simulink model "VIM_simu"  (R2022b)
settings: Solver=VariableStepAuto  StartTime=0.0  StopTime=0.7  MaxStep=1e-4  RelTol=1e-3
undefined symbols (not defined in the file or in its folder): motorParams, params_struct_torque
libraries: slpidlib x6, spsabctodq0Lib x6, spsdq0toabcLib x2, spsThreePhaseSeriesRLCBranchLib x2, spsThreePhaseSeriesRLCLoadLib x2, spsThreePhaseVIMeasurementLib x2, spsDCVoltageSourceLib x1, spsGroundLib x1, spsPower3phInstantaneousLib x1, spsPWMGenerator2LevelLib x1, spsThreePhaseBreakerLib x1, spsThreePhaseSourceLib x1
settings Model: Creator=Dong  LastModifiedBy=Dong
settings DebuggingCC: MaskedZcDiagnostic=none  IgnoredZcDiagnostic=none

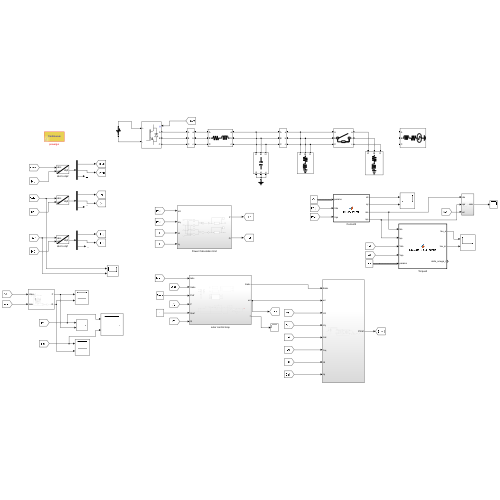
[thumbnail: Simulink's stored preview of the top-level diagram]
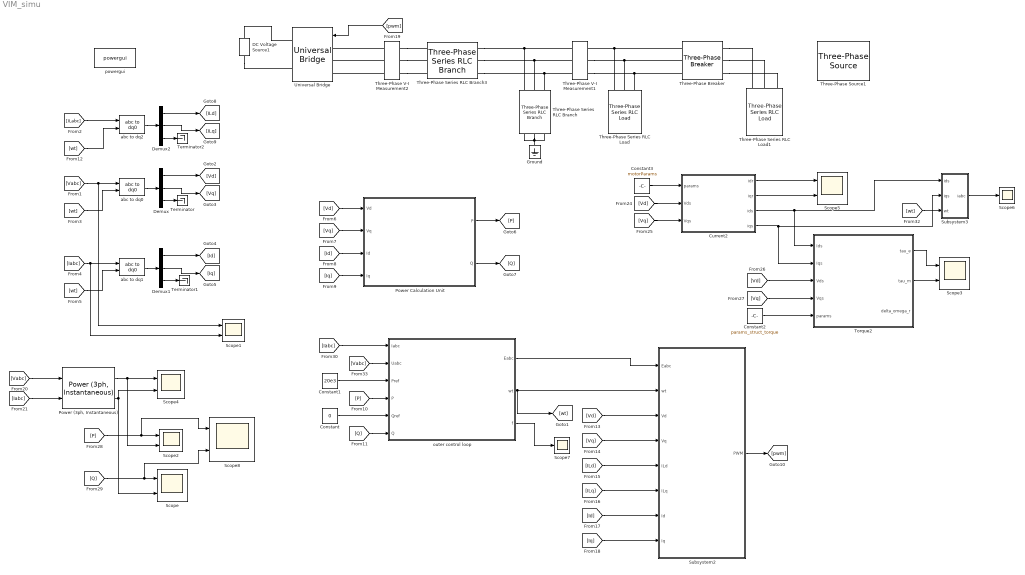
== system VIM_simu ==
  Constant : Constant  Value=0
  Constant1 : Constant  Value=20e3
  Constant2 : Constant  Value=params_struct_torque  OutDataTypeStr=Bus: paramsBusTorque
  Constant3 : Constant  Value=motorParams  OutDataTypeStr=Bus: motorParamsBus
  Current2 : MATLAB Function  TreatAsAtomicUnit=on
  DC Voltage Source1 : spsDCVoltageSourceLib/DC Voltage Source  Amplitude=800  Measurements=None
  Demux : Demux  Outputs=3
  Demux1 : Demux  Outputs=3
  Demux2 : Demux  Outputs=3
  Ground : spsGroundLib/Ground  LConnTagsString=a
  "Power (3ph, Instantaneous)" : spsPower3phInstantaneousLib/Power (3ph, Instantaneous)
  Power Calculation Unit : Subsystem
  Scope{,1..5,8} (7 alike) : Scope  NumInputPorts=2
  Scope6 : Scope
  Scope7 : Scope
  Subsystem2 : Subsystem
  Subsystem3 : Subsystem
  Terminator : Terminator
  Terminator1 : Terminator
  Terminator2 : Terminator
  Three-Phase Series RLC Branch : spsThreePhaseSeriesRLCBranchLib/Three-Phase Series RLC Branch  LConnTagsString=A|B|C  RConnTagsString=A|B|C  BranchType=C  Resistance=1e-5  Inductance=3e-3  Capacitance=40e-6  Measurements=None
  Three-Phase Series RLC Branch3 : spsThreePhaseSeriesRLCBranchLib/Three-Phase Series RLC Branch  LConnTagsString=A|B|C  RConnTagsString=A|B|C  BranchType=RL  Resistance=1e-5  Inductance=3e-3  Capacitance=1e-6  Measurements=None
  Three-Phase Series RLC Load : spsThreePhaseSeriesRLCLoadLib/Three-Phase Series RLC Load  LConnTagsString=A|B|C  Configuration=Y (grounded)  NominalVoltage=380  Vabc=[1e3 1e3 1e3]  Vabcp=[1e3 1e3 1e3]  NominalFrequency=50  UnbalancedPower=off  ActivePower=5e3  InductivePower=200  CapacitivePower=0  Pabc=[10e3 9e3 11e3]  QLabc=[100 90 110]  QCabc=[100 90 110]  Pabcp=[10e3 9e3 11e3]  QLabcp=[100 90 110]  QCabcp=[100 90 110]  Measurements=None  LoadType=constant Z
  Three-Phase Series RLC Load1 : spsThreePhaseSeriesRLCLoadLib/Three-Phase Series RLC Load  LConnTagsString=A|B|C  Configuration=Y (grounded)  NominalVoltage=380  Vabc=[1e3 1e3 1e3]  Vabcp=[1e3 1e3 1e3]  NominalFrequency=50  UnbalancedPower=off  ActivePower=5e3  InductivePower=500  CapacitivePower=0  Pabc=[10e3 9e3 11e3]  QLabc=[100 90 110]  QCabc=[100 90 110]  Pabcp=[10e3 9e3 11e3]  QLabcp=[100 90 110]  QCabcp=[100 90 110]  Measurements=None  LoadType=constant Z
  Three-Phase V-I Measurement1 : spsThreePhaseVIMeasurementLib/Three-Phase V-I Measurement  VoltageMeasurement=phase-to-ground  SetLabelV=on  LabelV=Vabc  Vpu=off  VpuLL=off  CurrentMeasurement=yes  SetLabelI=on  LabelI=Iabc  Ipu=off  Pbase=100e6  Vbase=500e3  OutputType=Complex  PhasorSimulation=off  PSBequivalent=0
  Three-Phase V-I Measurement2 : spsThreePhaseVIMeasurementLib/Three-Phase V-I Measurement  VoltageMeasurement=no  SetLabelV=off  LabelV=Vabc  Vpu=off  VpuLL=off  CurrentMeasurement=yes  SetLabelI=on  LabelI=ILabc  Ipu=off  Pbase=100e6  Vbase=500e3  OutputType=Complex  PhasorSimulation=off  PSBequivalent=0
  Three-Phase Breaker : spsThreePhaseBreakerLib/Three-Phase Breaker  InitialState=open  SwitchA=on  SwitchB=on  SwitchC=on  SwitchTimes=[0.1 0.4]  External=off  BreakerResistance=0.01  SnubberResistance=1e6  SnubberCapacitance=inf  Measurements=None
  Three-Phase Source1 : spsThreePhaseSourceLib/Three-Phase Source  InternalConnection=Yg  VoltagePhases=off  Voltage=380  PhaseAngle=0  Voltage_phases=[25e3 25e3 25e3]/sqrt(3)  PhaseAngles_phases=[0 -120 +120]  Frequency=50  NonIdealSource=on  SpecifyImpedance=off  Resistance=1e-4  Inductance=1e-3  ShortCircuitLevel=100e6  BaseVoltage=25e3  XRratio=7  BusType=swing  Pref=10e3  Qref=0  Prefabc=[10e3, 10e3, 10e3]  Qrefabc=[0, 0, 0]  Qmin=-inf  Qmax=inf
  Torque2 : MATLAB Function  TreatAsAtomicUnit=on
  Universal Bridge : spsUniversalBridgeLib/Universal Bridge  Arms=3  SnubberResistance=1e5  SnubberCapacitance=inf  Device=IGBT / Diodes  Ron=1e-3  Lon=0  ForwardVoltages="[  0  0  ]"  ForwardVoltage=0  GTOparameters=[ 10e-6 , 20e-6 ]  IGBTparameters=[ 1e-6 , 2e-6 ]  Measurements=None  Measurements_2=None  converterType=Rectifier
  abc to dq0 : spsabctodq0Lib/abc to dq0  Alignment=90 degrees behind phase A axis
  abc to dq1 : spsabctodq0Lib/abc to dq0  Alignment=90 degrees behind phase A axis
  abc to dq2 : spsabctodq0Lib/abc to dq0  Alignment=90 degrees behind phase A axis
  outer control loop : Subsystem
  powergui : sps_lib/powergui  Priority=1  SimulationMode=Continuous  SampleTime=50e-6  frequency=60  Iterations=50  frequencyindice=0  Pbase=100e6  ErrMax=1e-4  UnitsV=kV  UnitsW=MW  buscounter=0  FunctionMessages=off  echomessages=off  EnableUseOfTLC=off  CurrentSourceSwitches=off  DisableSnubberDevices=off  DisableRonSwitches=off  DisableVfSwitches=off  DisplayEquations=off  AutomaticDiscreteSolvers=off  SolverType=Tustin/Backward Euler (TBE)  Interpol=off  ExternalGateDelay=off  methode=off  Ts=100  x0status=blocks  SPID=on  SwTol=0  HookPort=off  NonlinearTolerance=1e-4  nMaxIteration=100  ContinueOnMaxIteration=off  RestoreLinks=warning  ResistiveCurrentMeasurement=off  Frange=[0:2:500]  Ylog=off  Xlog=on  ShowGrid=off  save=off  variable=ZData  structure=0  ZoomFFT=off  StartTime=0.0  cycles=1  DisplayStyle=1  fundamental=60  FreqAxis=off  MaxFrequency=1000  frequencyindicesteady=1  RmsSteady=1  display=off
  wires:
  Constant/1 -> outer control loop/5(Qref)
  Constant1/1 -> outer control loop/3(Pref)
  [Vabc] -> abc to dq0/1, Scope1/1
  [wt] -> abc to dq0/2
  [wt] -> abc to dq1/2
  [Iabc] -> Scope1/2, abc to dq1/1
  abc to dq0/1 -> Demux/1
  abc to dq1/1 -> Demux1/1
  Demux1/3 -> Terminator1/1
  Demux/3 -> Terminator/1
  Demux/1 -> [Vd]
  Demux/2 -> [Vq]
  Demux1/2 -> [Iq]
  Demux1/1 -> [Id]
  [Vd] -> Power Calculation Unit/1(Vd)
  [Vq] -> Power Calculation Unit/2(Vq)
  [Id] -> Power Calculation Unit/3(Id)
  [Iq] -> Power Calculation Unit/4(Iq)
  Power Calculation Unit/1(P) -> [P]
  Power Calculation Unit/2(Q) -> [Q]
  [P] -> outer control loop/4(P)
  [Q] -> outer control loop/6(Q)
  Demux2/2 -> [ILq]
  Demux2/1 -> [ILd]
  Demux2/3 -> Terminator2/1
  abc to dq2/1 -> Demux2/1
  [wt] -> abc to dq2/2
  [ILabc] -> abc to dq2/1
  outer control loop/1(Eabc) -> Subsystem2/1(Eabc)
  [Vd] -> Subsystem2/3(Vd)
  [Vq] -> Subsystem2/4(Vq)
  [ILd] -> Subsystem2/5(ILd)
  [ILq] -> Subsystem2/6(ILq)
  [Iq] -> Subsystem2/8(Iq)
  [Id] -> Subsystem2/7(Id)
  Subsystem2/1(PWM) -> [pwm]
  [pwm] -> Universal Bridge/1
  outer control loop/2(wt) -> [wt], Subsystem2/2(wt)
  [Vabc] -> "Power (3ph, Instantaneous)"/1
  [Iabc] -> "Power (3ph, Instantaneous)"/2
  "Power (3ph, Instantaneous)"/1 -> Scope2/2, Scope4/1
  "Power (3ph, Instantaneous)"/2 -> Scope/2, Scope4/2
  Constant3/1 -> Current2/1(params)
  Constant2/1 -> Torque2/5(params)
  Current2/3(ids) -> Subsystem3/1(ids), Torque2/1(Ids)
  Current2/4(iqs) -> Torque2/2(Iqs), Subsystem3/2(iqs)
  [Vq] -> Current2/3(Vqs)
  [Vd] -> Current2/2(Vds)
  [Vq] -> Torque2/4(Vqs)
  [Vd] -> Torque2/3(Vds)
  Torque2/1(tau_e) -> Scope3/1
  Torque2/2(tau_m) -> Scope3/2
  Current2/1(idr) -> Scope5/1
  Current2/2(iqr) -> Scope5/2
  [P] -> Scope8/1, Scope2/1
  [Q] -> Scope8/2, Scope/1
  [wt] -> Subsystem3/3(wt)
  Subsystem3/1(iabc) -> Scope6/1
  outer control loop/3(f) -> Scope7/1
  [Vabc] -> outer control loop/2(Uabc)
  [Iabc] -> outer control loop/1(Iabc)
  connections:
  Three-Phase Breaker/RConn2 -- Three-Phase Series RLC Load1/LConn2
  Three-Phase Series RLC Branch/LConn3 -- Three-Phase Series RLC Branch3/RConn3 -- Three-Phase V-I Measurement1/LConn3
  Three-Phase Series RLC Branch/LConn2 -- Three-Phase Series RLC Branch3/RConn2 -- Three-Phase V-I Measurement1/LConn2
  Three-Phase Series RLC Branch/LConn1 -- Three-Phase Series RLC Branch3/RConn1 -- Three-Phase V-I Measurement1/LConn1
  DC Voltage Source1/RConn1 -- Universal Bridge/RConn1
  DC Voltage Source1/LConn1 -- Universal Bridge/RConn2
  Three-Phase Breaker/RConn1 -- Three-Phase Series RLC Load1/LConn1
  Three-Phase Breaker/RConn3 -- Three-Phase Series RLC Load1/LConn3
  Three-Phase Series RLC Branch/RConn1 -- Ground/LConn1 -- Three-Phase Series RLC Branch/RConn2 -- Three-Phase Series RLC Branch/RConn3
  Three-Phase Breaker/LConn1 -- Three-Phase V-I Measurement1/RConn1 -- Three-Phase Series RLC Load/LConn1
  Three-Phase V-I Measurement1/RConn2 -- Three-Phase Breaker/LConn2 -- Three-Phase Series RLC Load/LConn2
  Three-Phase V-I Measurement1/RConn3 -- Three-Phase Breaker/LConn3 -- Three-Phase Series RLC Load/LConn3
  Three-Phase V-I Measurement2/RConn1 -- Three-Phase Series RLC Branch3/LConn1
  Three-Phase V-I Measurement2/RConn2 -- Three-Phase Series RLC Branch3/LConn2
  Three-Phase V-I Measurement2/RConn3 -- Three-Phase Series RLC Branch3/LConn3
  Three-Phase V-I Measurement2/LConn3 -- Universal Bridge/LConn3
  Three-Phase V-I Measurement2/LConn2 -- Universal Bridge/LConn2
  Three-Phase V-I Measurement2/LConn1 -- Universal Bridge/LConn1

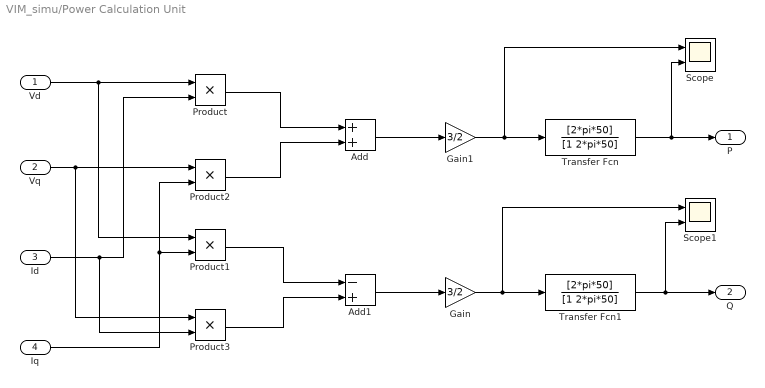
== system VIM_simu/Power Calculation Unit ==
  Vd : Inport
  Vq : Inport  Port=2
  Id : Inport  Port=3
  Iq : Inport  Port=4
  Add : Sum
  Add1 : Sum  Inputs=-+
  Gain : Gain  Gain=3/2
  Gain1 : Gain  Gain=3/2
  Product{,1..3} (4 alike) : Product
  Scope : Scope  NumInputPorts=2
  Scope1 : Scope  NumInputPorts=2
  Transfer Fcn : TransferFcn  Numerator=[2*pi*50]  Denominator=[1 2*pi*50]
  Transfer Fcn1 : TransferFcn  Numerator=[2*pi*50]  Denominator=[1 2*pi*50]
  P : Outport
  Q : Outport  Port=2
  wires:
  Vd/1 -> Product1/1, Product/1
  Vq/1 -> Product3/1, Product2/1
  Id/1 -> Product3/2, Product/2
  Iq/1 -> Product1/2, Product2/2
  Product3/1 -> Add1/2
  Product/1 -> Add/1
  Product2/1 -> Add/2
  Add1/1 -> Gain/1
  Add/1 -> Gain1/1
  Gain1/1 -> Scope/1, Transfer Fcn/1
  Transfer Fcn/1 -> Scope/2, P/1
  Transfer Fcn1/1 -> Scope1/2, Q/1
  Gain/1 -> Scope1/1, Transfer Fcn1/1
  Product1/1 -> Add1/1

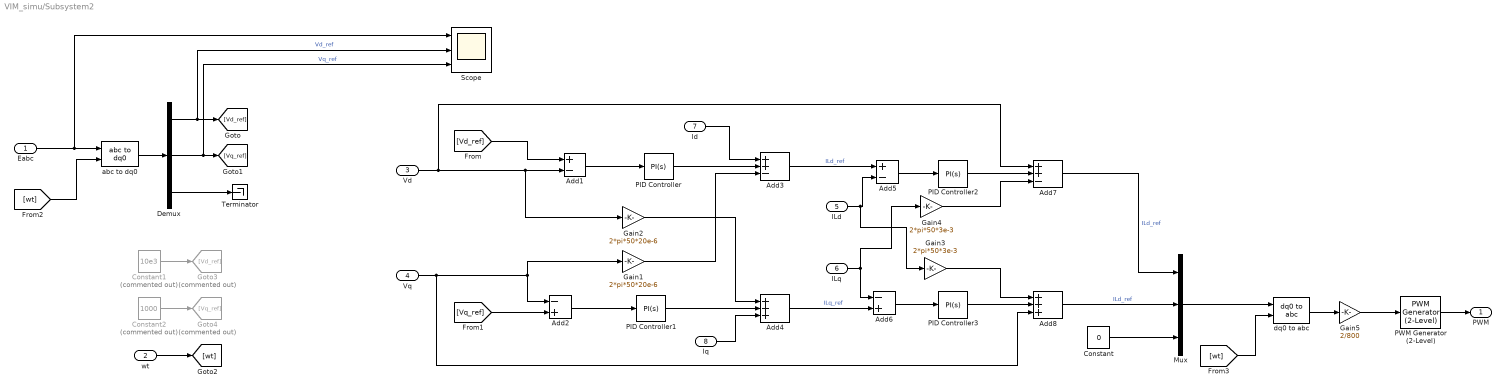
== system VIM_simu/Subsystem2 ==
  Eabc : Inport
  wt : Inport  Port=2
  Vd : Inport  Port=3
  Vq : Inport  Port=4
  ILd : Inport  Port=5
  ILq : Inport  Port=6
  Id : Inport  Port=7
  Iq : Inport  Port=8
  Add1 : Sum  Inputs=+-
  Add2 : Sum  Inputs=-+
  Add3 : Sum  Inputs=++-
  Add4 : Sum  Inputs=+++
  Add5 : Sum  Inputs=+-
  Add6 : Sum  Inputs=-+
  Add7 : Sum  Inputs=++-
  Add8 : Sum  Inputs=+++
  Constant : Constant  Value=0
  Constant1 : Constant  Commented=on  Value=10e3
  Constant2 : Constant  Commented=on  Value=1000
  Demux : Demux  Outputs=3
  Gain1 : Gain  Gain=2*pi*50*20e-6
  Gain2 : Gain  Gain=2*pi*50*20e-6
  Gain3 : Gain  Gain=2*pi*50*3e-3
  Gain4 : Gain  Gain=2*pi*50*3e-3
  Gain5 : Gain  Gain=2/800
  Goto3 : Goto  Commented=on  GotoTag=Vd_ref
  Goto4 : Goto  Commented=on  GotoTag=Vq_ref
  Mux : Mux  Inputs=3
  PID Controller : slpidlib/PID Controller  Controller=PI  Form=Parallel  TimeDomain=Continuous-time  UseExternalTs=off  SampleTime=-1  IntegratorMethod=Forward Euler  FilterMethod=Forward Euler  ControllerParametersSource=internal  P=0.5  I=10  UseKiTs=off  D=0  N=100  UseFilter=on  TunerSelectOption=Transfer Function Based (PID Tuner App)  InitialConditionSource=internal  InitialConditionForIntegrator=0  InitialConditionForFilter=0  DifferentiatorICPrevScaledInput=0  ExternalReset=none  TrackingMode=off  Kt=1  LimitOutput=off  SatLimitsSource=internal  UpperSaturationLimit=inf  LowerSaturationLimit=-inf  LinearizeAsGain=on  AntiWindupMode=none  Kb=1  LimitIntegrator=off  UpperIntegratorSaturationLimit=inf  LowerIntegratorSaturationLimit=-inf  POutMin=[]  POutMax=[]  IOutMin=[]  IOutMax=[]  DOutMin=[]  DOutMax=[]  NOutMin=[]  NOutMax=[]  SumOutMin=[]  SumOutMax=[]  SaturationOutMin=[]  SaturationOutMax=[]  PParamMin=[]  PParamMax=[]  IParamMin=[]  IParamMax=[]  DParamMin=[]  DParamMax=[]  NParamMin=[]  NParamMax=[]  KbParamMin=[]  KbParamMax=[]  KtParamMin=[]  KtParamMax=[]  KbOutMin=[]  KbOutMax=[]  KtOutMin=[]  KtOutMax=[]  IntegratorOutMin=[]  IntegratorOutMax=[]  FilterOutMin=[]  FilterOutMax=[]  SumI1OutMin=[]  SumI1OutMax=[]  SumI2OutMin=[]  SumI2OutMax=[]  SumI3OutMin=[]  SumI3OutMax=[]  SumI4OutMin=[]  SumI4OutMax=[]  SumDOutMin=[]  SumDOutMax=[]  DifferentiatorOutMin=[]  DifferentiatorOutMax=[]  FilterDiffOutCoefMin=[]  FilterDiffOutCoefMax=[]  ReciprocalOutMin=[]  ReciprocalOutMax=[]  SumDenOutMin=[]  SumDenOutMax=[]  SumNumOutMin=[]  SumNumOutMax=[]  DivideOutMin=[]  DivideOutMax=[]  UdiffTsProdOutMin=[]  UdiffTsProdOutMax=[]  NTsProdOutMin=[]  NTsProdOutMax=[]  UintegralTsProdOutMin=[]  UintegralTsProdOutMax=[]  UngainTsProdOutMin=[]  UngainTsProdOutMax=[]  ClampingZeroOutDataTypeStr=Inherit: Inherit via back propagation  ClampingZeroOutMin=[]  ClampingZeroOutMax=[]  FilterDenConstantOutDataTypeStr=Inherit: Inherit via back propagation  FilterDenConstantOutMin=[]  FilterDenConstantOutMax=[]  PCopyOutDataTypeStr=Inherit: Inherit via back propagation  PCopyOutMin=[]  PCopyOutMax=[]  NCopyOutDataTypeStr=Inherit: Inherit via back propagation  NCopyOutMin=[]  NCopyOutMax=[]  IntegratorContinuousStateAttributes=''  IntegratorStateMustResolveToSignalObject=off  IntegratorRTWStateStorageClass=Auto  FilterContinuousStateAttributes=''  FilterStateMustResolveToSignalObject=off  FilterRTWStateStorageClass=Auto  ParallelPVariant=InternalParameters  IdealPVariant=Disabled  IVariant=InternalParameters  DVariant=Disabled  IntegratorVariant=Continuous  SatVariant=Disabled  AWVariant=Passthrough  PCopyVariant=Disabled  TRVariant=Disabled  FdbkBlocksVariant=Forward  IdealPFdbkVariant=Disabled  SatFdbkVariant=Disabled  DerivativeFilterVariant=Disabled  NVariant=Disabled  NCopyVariant=Disabled_SignalSpec  FilterICVariant=Disabled  IntegratorICVariant=InternalICs  ExternalResetVariant=Disabled  TRSumVariant=Passthrough  SumFdbkVariant=Disabled  SumVariant=Sum_PI  TsampFilterVariant=InternalTs  TsampNgainVariant=Passthrough  TsampIntegralVariant=Passthrough  ExternalSaturationOutDataTypeStr=Inherit: Same as second input
  PID Controller1 : slpidlib/PID Controller  Controller=PI  Form=Parallel  TimeDomain=Continuous-time  UseExternalTs=off  SampleTime=-1  IntegratorMethod=Forward Euler  FilterMethod=Forward Euler  ControllerParametersSource=internal  P=0.5  I=10  UseKiTs=off  D=0  N=100  UseFilter=on  TunerSelectOption=Transfer Function Based (PID Tuner App)  InitialConditionSource=internal  InitialConditionForIntegrator=0  InitialConditionForFilter=0  DifferentiatorICPrevScaledInput=0  ExternalReset=none  TrackingMode=off  Kt=1  LimitOutput=off  SatLimitsSource=internal  UpperSaturationLimit=inf  LowerSaturationLimit=-inf  LinearizeAsGain=on  AntiWindupMode=none  Kb=1  LimitIntegrator=off  UpperIntegratorSaturationLimit=inf  LowerIntegratorSaturationLimit=-inf  POutMin=[]  POutMax=[]  IOutMin=[]  IOutMax=[]  DOutMin=[]  DOutMax=[]  NOutMin=[]  NOutMax=[]  SumOutMin=[]  SumOutMax=[]  SaturationOutMin=[]  SaturationOutMax=[]  PParamMin=[]  PParamMax=[]  IParamMin=[]  IParamMax=[]  DParamMin=[]  DParamMax=[]  NParamMin=[]  NParamMax=[]  KbParamMin=[]  KbParamMax=[]  KtParamMin=[]  KtParamMax=[]  KbOutMin=[]  KbOutMax=[]  KtOutMin=[]  KtOutMax=[]  IntegratorOutMin=[]  IntegratorOutMax=[]  FilterOutMin=[]  FilterOutMax=[]  SumI1OutMin=[]  SumI1OutMax=[]  SumI2OutMin=[]  SumI2OutMax=[]  SumI3OutMin=[]  SumI3OutMax=[]  SumI4OutMin=[]  SumI4OutMax=[]  SumDOutMin=[]  SumDOutMax=[]  DifferentiatorOutMin=[]  DifferentiatorOutMax=[]  FilterDiffOutCoefMin=[]  FilterDiffOutCoefMax=[]  ReciprocalOutMin=[]  ReciprocalOutMax=[]  SumDenOutMin=[]  SumDenOutMax=[]  SumNumOutMin=[]  SumNumOutMax=[]  DivideOutMin=[]  DivideOutMax=[]  UdiffTsProdOutMin=[]  UdiffTsProdOutMax=[]  NTsProdOutMin=[]  NTsProdOutMax=[]  UintegralTsProdOutMin=[]  UintegralTsProdOutMax=[]  UngainTsProdOutMin=[]  UngainTsProdOutMax=[]  ClampingZeroOutDataTypeStr=Inherit: Inherit via back propagation  ClampingZeroOutMin=[]  ClampingZeroOutMax=[]  FilterDenConstantOutDataTypeStr=Inherit: Inherit via back propagation  FilterDenConstantOutMin=[]  FilterDenConstantOutMax=[]  PCopyOutDataTypeStr=Inherit: Inherit via back propagation  PCopyOutMin=[]  PCopyOutMax=[]  NCopyOutDataTypeStr=Inherit: Inherit via back propagation  NCopyOutMin=[]  NCopyOutMax=[]  IntegratorContinuousStateAttributes=''  IntegratorStateMustResolveToSignalObject=off  IntegratorRTWStateStorageClass=Auto  FilterContinuousStateAttributes=''  FilterStateMustResolveToSignalObject=off  FilterRTWStateStorageClass=Auto  ParallelPVariant=InternalParameters  IdealPVariant=Disabled  IVariant=InternalParameters  DVariant=Disabled  IntegratorVariant=Continuous  SatVariant=Disabled  AWVariant=Passthrough  PCopyVariant=Disabled  TRVariant=Disabled  FdbkBlocksVariant=Forward  IdealPFdbkVariant=Disabled  SatFdbkVariant=Disabled  DerivativeFilterVariant=Disabled  NVariant=Disabled  NCopyVariant=Disabled_SignalSpec  FilterICVariant=Disabled  IntegratorICVariant=InternalICs  ExternalResetVariant=Disabled  TRSumVariant=Passthrough  SumFdbkVariant=Disabled  SumVariant=Sum_PI  TsampFilterVariant=InternalTs  TsampNgainVariant=Passthrough  TsampIntegralVariant=Passthrough  ExternalSaturationOutDataTypeStr=Inherit: Same as second input
  PID Controller2 : slpidlib/PID Controller  Controller=PI  Form=Parallel  TimeDomain=Continuous-time  UseExternalTs=off  SampleTime=-1  IntegratorMethod=Forward Euler  FilterMethod=Forward Euler  ControllerParametersSource=internal  P=50  I=100  UseKiTs=off  D=0  N=100  UseFilter=on  TunerSelectOption=Transfer Function Based (PID Tuner App)  InitialConditionSource=internal  InitialConditionForIntegrator=0  InitialConditionForFilter=0  DifferentiatorICPrevScaledInput=0  ExternalReset=none  TrackingMode=off  Kt=1  LimitOutput=off  SatLimitsSource=internal  UpperSaturationLimit=inf  LowerSaturationLimit=-inf  LinearizeAsGain=on  AntiWindupMode=none  Kb=1  LimitIntegrator=off  UpperIntegratorSaturationLimit=inf  LowerIntegratorSaturationLimit=-inf  POutMin=[]  POutMax=[]  IOutMin=[]  IOutMax=[]  DOutMin=[]  DOutMax=[]  NOutMin=[]  NOutMax=[]  SumOutMin=[]  SumOutMax=[]  SaturationOutMin=[]  SaturationOutMax=[]  PParamMin=[]  PParamMax=[]  IParamMin=[]  IParamMax=[]  DParamMin=[]  DParamMax=[]  NParamMin=[]  NParamMax=[]  KbParamMin=[]  KbParamMax=[]  KtParamMin=[]  KtParamMax=[]  KbOutMin=[]  KbOutMax=[]  KtOutMin=[]  KtOutMax=[]  IntegratorOutMin=[]  IntegratorOutMax=[]  FilterOutMin=[]  FilterOutMax=[]  SumI1OutMin=[]  SumI1OutMax=[]  SumI2OutMin=[]  SumI2OutMax=[]  SumI3OutMin=[]  SumI3OutMax=[]  SumI4OutMin=[]  SumI4OutMax=[]  SumDOutMin=[]  SumDOutMax=[]  DifferentiatorOutMin=[]  DifferentiatorOutMax=[]  FilterDiffOutCoefMin=[]  FilterDiffOutCoefMax=[]  ReciprocalOutMin=[]  ReciprocalOutMax=[]  SumDenOutMin=[]  SumDenOutMax=[]  SumNumOutMin=[]  SumNumOutMax=[]  DivideOutMin=[]  DivideOutMax=[]  UdiffTsProdOutMin=[]  UdiffTsProdOutMax=[]  NTsProdOutMin=[]  NTsProdOutMax=[]  UintegralTsProdOutMin=[]  UintegralTsProdOutMax=[]  UngainTsProdOutMin=[]  UngainTsProdOutMax=[]  ClampingZeroOutDataTypeStr=Inherit: Inherit via back propagation  ClampingZeroOutMin=[]  ClampingZeroOutMax=[]  FilterDenConstantOutDataTypeStr=Inherit: Inherit via back propagation  FilterDenConstantOutMin=[]  FilterDenConstantOutMax=[]  PCopyOutDataTypeStr=Inherit: Inherit via back propagation  PCopyOutMin=[]  PCopyOutMax=[]  NCopyOutDataTypeStr=Inherit: Inherit via back propagation  NCopyOutMin=[]  NCopyOutMax=[]  IntegratorContinuousStateAttributes=''  IntegratorStateMustResolveToSignalObject=off  IntegratorRTWStateStorageClass=Auto  FilterContinuousStateAttributes=''  FilterStateMustResolveToSignalObject=off  FilterRTWStateStorageClass=Auto  ParallelPVariant=InternalParameters  IdealPVariant=Disabled  IVariant=InternalParameters  DVariant=Disabled  IntegratorVariant=Continuous  SatVariant=Disabled  AWVariant=Passthrough  PCopyVariant=Disabled  TRVariant=Disabled  FdbkBlocksVariant=Forward  IdealPFdbkVariant=Disabled  SatFdbkVariant=Disabled  DerivativeFilterVariant=Disabled  NVariant=Disabled  NCopyVariant=Disabled_SignalSpec  FilterICVariant=Disabled  IntegratorICVariant=InternalICs  ExternalResetVariant=Disabled  TRSumVariant=Passthrough  SumFdbkVariant=Disabled  SumVariant=Sum_PI  TsampFilterVariant=InternalTs  TsampNgainVariant=Passthrough  TsampIntegralVariant=Passthrough  ExternalSaturationOutDataTypeStr=Inherit: Same as second input
  PID Controller3 : slpidlib/PID Controller  Controller=PI  Form=Parallel  TimeDomain=Continuous-time  UseExternalTs=off  SampleTime=-1  IntegratorMethod=Forward Euler  FilterMethod=Forward Euler  ControllerParametersSource=internal  P=0.5  I=10  UseKiTs=off  D=0  N=100  UseFilter=on  TunerSelectOption=Transfer Function Based (PID Tuner App)  InitialConditionSource=internal  InitialConditionForIntegrator=0  InitialConditionForFilter=0  DifferentiatorICPrevScaledInput=0  ExternalReset=none  TrackingMode=off  Kt=1  LimitOutput=off  SatLimitsSource=internal  UpperSaturationLimit=inf  LowerSaturationLimit=-inf  LinearizeAsGain=on  AntiWindupMode=none  Kb=1  LimitIntegrator=off  UpperIntegratorSaturationLimit=inf  LowerIntegratorSaturationLimit=-inf  POutMin=[]  POutMax=[]  IOutMin=[]  IOutMax=[]  DOutMin=[]  DOutMax=[]  NOutMin=[]  NOutMax=[]  SumOutMin=[]  SumOutMax=[]  SaturationOutMin=[]  SaturationOutMax=[]  PParamMin=[]  PParamMax=[]  IParamMin=[]  IParamMax=[]  DParamMin=[]  DParamMax=[]  NParamMin=[]  NParamMax=[]  KbParamMin=[]  KbParamMax=[]  KtParamMin=[]  KtParamMax=[]  KbOutMin=[]  KbOutMax=[]  KtOutMin=[]  KtOutMax=[]  IntegratorOutMin=[]  IntegratorOutMax=[]  FilterOutMin=[]  FilterOutMax=[]  SumI1OutMin=[]  SumI1OutMax=[]  SumI2OutMin=[]  SumI2OutMax=[]  SumI3OutMin=[]  SumI3OutMax=[]  SumI4OutMin=[]  SumI4OutMax=[]  SumDOutMin=[]  SumDOutMax=[]  DifferentiatorOutMin=[]  DifferentiatorOutMax=[]  FilterDiffOutCoefMin=[]  FilterDiffOutCoefMax=[]  ReciprocalOutMin=[]  ReciprocalOutMax=[]  SumDenOutMin=[]  SumDenOutMax=[]  SumNumOutMin=[]  SumNumOutMax=[]  DivideOutMin=[]  DivideOutMax=[]  UdiffTsProdOutMin=[]  UdiffTsProdOutMax=[]  NTsProdOutMin=[]  NTsProdOutMax=[]  UintegralTsProdOutMin=[]  UintegralTsProdOutMax=[]  UngainTsProdOutMin=[]  UngainTsProdOutMax=[]  ClampingZeroOutDataTypeStr=Inherit: Inherit via back propagation  ClampingZeroOutMin=[]  ClampingZeroOutMax=[]  FilterDenConstantOutDataTypeStr=Inherit: Inherit via back propagation  FilterDenConstantOutMin=[]  FilterDenConstantOutMax=[]  PCopyOutDataTypeStr=Inherit: Inherit via back propagation  PCopyOutMin=[]  PCopyOutMax=[]  NCopyOutDataTypeStr=Inherit: Inherit via back propagation  NCopyOutMin=[]  NCopyOutMax=[]  IntegratorContinuousStateAttributes=''  IntegratorStateMustResolveToSignalObject=off  IntegratorRTWStateStorageClass=Auto  FilterContinuousStateAttributes=''  FilterStateMustResolveToSignalObject=off  FilterRTWStateStorageClass=Auto  ParallelPVariant=InternalParameters  IdealPVariant=Disabled  IVariant=InternalParameters  DVariant=Disabled  IntegratorVariant=Continuous  SatVariant=Disabled  AWVariant=Passthrough  PCopyVariant=Disabled  TRVariant=Disabled  FdbkBlocksVariant=Forward  IdealPFdbkVariant=Disabled  SatFdbkVariant=Disabled  DerivativeFilterVariant=Disabled  NVariant=Disabled  NCopyVariant=Disabled_SignalSpec  FilterICVariant=Disabled  IntegratorICVariant=InternalICs  ExternalResetVariant=Disabled  TRSumVariant=Passthrough  SumFdbkVariant=Disabled  SumVariant=Sum_PI  TsampFilterVariant=InternalTs  TsampNgainVariant=Passthrough  TsampIntegralVariant=Passthrough  ExternalSaturationOutDataTypeStr=Inherit: Same as second input
  PWM Generator (2-Level) : spsPWMGenerator2LevelLib/PWM Generator (2-Level)  ModulatorType=Three-phase bridge (6 pulses)  ModulatorMode=Unsynchronized  Fc=10e3  Pc=90  nF=27  MinMax="[ -1  1 ]"  SamplingTechnique=Natural  ModulatingSignals=off  m=0.8  Freq=60  Phase=0  Ts=0  ShowCarrierOutport=off
  Scope : Scope  NumInputPorts=3
  Terminator : Terminator
  abc to dq0 : spsabctodq0Lib/abc to dq0  Alignment=90 degrees behind phase A axis
  dq0 to abc : spsdq0toabcLib/dq0 to abc  Alignment=90 degrees behind phase A axis
  PWM : Outport
  wires:
  Eabc/1 -> Scope/1, abc to dq0/1
  Demux/3 -> Terminator/1
  Add1/1 -> PID Controller/1
  Add2/1 -> PID Controller1/1
  Id/1 -> Add3/1
  PID Controller/1 -> Add3/2
  Gain1/1 -> Add3/3
  Vq/1 -> Add8/3, Add2/1, Gain1/1
  Vd/1 -> Add7/1, Gain2/1, Add1/2
  PID Controller1/1 -> Add4/2
  Iq/1 -> Add4/3
  Gain2/1 -> Add4/1
  Demux/1 -> Scope/2, [Vd_ref]  "Vd_ref"
  abc to dq0/1 -> Demux/1
  Demux/2 -> Scope/3, [Vq_ref]  "Vq_ref"
  [Vq_ref] -> Add2/2
  [Vd_ref] -> Add1/1
  ILd/1 -> Gain3/1, Add5/2
  Add3/1 -> Add5/1  "ILd_ref"
  Add5/1 -> PID Controller2/1
  Add6/1 -> PID Controller3/1
  PID Controller3/1 -> Add8/2
  PID Controller2/1 -> Add7/2
  Add4/1 -> Add6/2  "ILq_ref"
  ILq/1 -> Gain4/1, Add6/1
  Gain3/1 -> Add8/1
  Gain4/1 -> Add7/3
  Constant/1 -> Mux/3
  Add8/1 -> Mux/2  "ILd_ref"
  Add7/1 -> Mux/1  "ILd_ref"
  Mux/1 -> dq0 to abc/1
  wt/1 -> [wt]
  [wt] -> abc to dq0/2
  [wt] -> dq0 to abc/2
  dq0 to abc/1 -> Gain5/1
  Gain5/1 -> PWM Generator (2-Level)/1
  PWM Generator (2-Level)/1 -> PWM/1
  Constant1/1 -> Goto3/1
  Constant2/1 -> Goto4/1

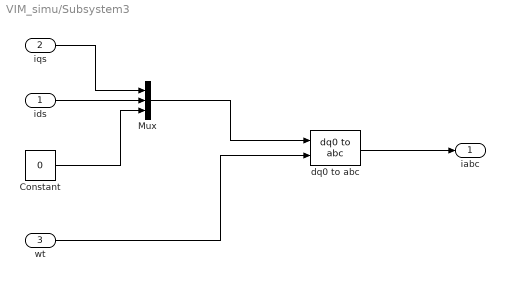
== system VIM_simu/Subsystem3 ==
  ids : Inport
  iqs : Inport  Port=2
  wt : Inport  Port=3
  Constant : Constant  Value=0
  Mux : Mux  Inputs=3
  dq0 to abc : spsdq0toabcLib/dq0 to abc  Alignment=90 degrees behind phase A axis
  iabc : Outport
  wires:
  Constant/1 -> Mux/3
  ids/1 -> Mux/2
  iqs/1 -> Mux/1
  Mux/1 -> dq0 to abc/1
  wt/1 -> dq0 to abc/2
  dq0 to abc/1 -> iabc/1

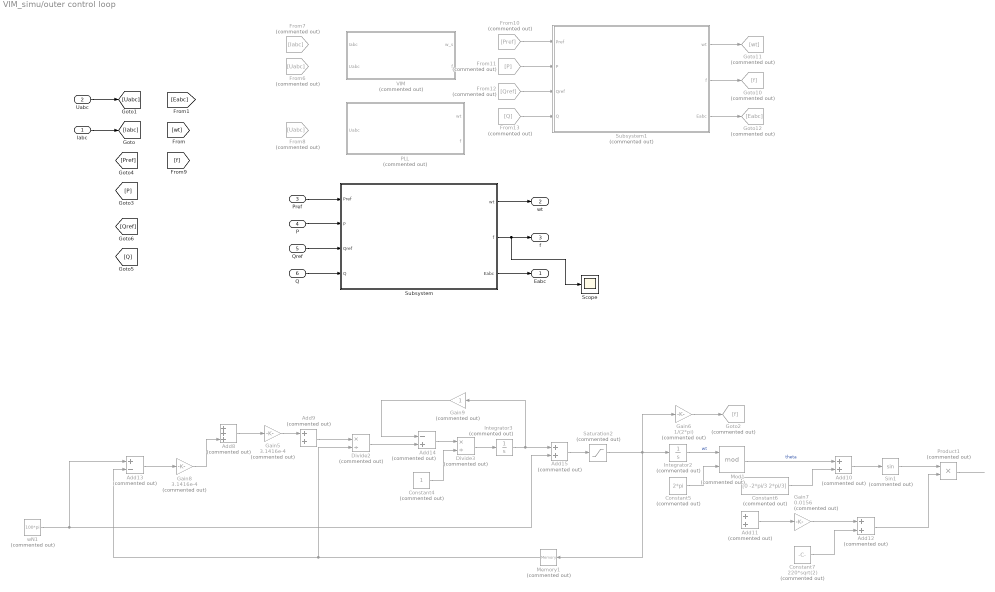
== system VIM_simu/outer control loop ==
  Iabc : Inport
  Uabc : Inport  Port=2
  Pref : Inport  Port=3
  P : Inport  Port=4
  Qref : Inport  Port=5
  Q : Inport  Port=6
  Add{9..12,15} (5 alike) : Sum  Commented=on
  Add13 : Sum  Commented=on  Inputs=+-
  Add14 : Sum  Commented=on  Inputs=-+
  Add8 : Sum  Commented=on  Inputs=+++
  Constant4 : Constant  Commented=on
  Constant5 : Constant  Commented=on  Value=2*pi
  Constant6 : Constant  Commented=on  Value=[0 -2*pi/3 2*pi/3]
  Constant7 : Constant  Commented=on  Value=220*sqrt(2)
  Divide2 : Product  Commented=on  Inputs=*/
  Divide3 : Product  Commented=on  Inputs=*/
  From10 : From  Commented=on  GotoTag=Pref
  From11 : From  Commented=on  GotoTag=P
  From12 : From  Commented=on  GotoTag=Qref
  From13 : From  Commented=on  GotoTag=Q
  From6 : From  Commented=on  GotoTag=Uabc
  From7 : From  Commented=on  GotoTag=Iabc
  From8 : From  Commented=on  GotoTag=Uabc
  Gain5 : Gain  Commented=on  Gain=3.1416e-4
  Gain6 : Gain  Commented=on  Gain=1/(2*pi)
  Gain7 : Gain  Commented=on  Gain=0.0156
  Gain8 : Gain  Commented=on  Gain=3.1416e-4
  Gain9 : Gain  Commented=on
  Goto10 : Goto  Commented=on  GotoTag=f
  Goto11 : Goto  Commented=on  GotoTag=wt
  Goto12 : Goto  Commented=on  GotoTag=Eabc
  Goto2 : Goto  Commented=on  GotoTag=f
  Integrator2 : Integrator  Commented=on
  Integrator3 : Integrator  Commented=on
  Memory1 : Memory  Commented=on  InitialCondition=2*pi*50
  Mod1 : Math  Commented=on  Operator=mod
  PLL : Subsystem  Commented=on
  Product1 : Product  Commented=on
  Saturation2 : Saturate  Commented=on  UpperLimit=1  LowerLimit=-1
  Scope : Scope
  Sin1 : Trigonometry  Commented=on
  Subsystem : Subsystem
  Subsystem1 : Subsystem  Commented=on
  VIM : Subsystem  Commented=on
  wN1 : Constant  Commented=on  Value=100*pi
  Eabc : Outport
  wt : Outport  Port=2
  f : Outport  Port=3
  wires:
  Divide3/1 -> Integrator3/1
  Add14/1 -> Divide3/1
  Constant4/1 -> Divide3/2
  Memory1/1 -> Add13/2, Divide2/2
  Gain9/1 -> Add14/1
  Constant7/1 -> Add12/2
  Add15/1 -> Saturation2/1
  Add10/1 -> Sin1/1
  Add9/1 -> Divide2/1
  Add8/1 -> Gain5/1
  Add11/1 -> Gain7/1
  Product1/1 -> ?
  Mod1/1 -> Add10/1  "theta"
  Gain7/1 -> Add12/1
  Gain5/1 -> Add9/1
  Saturation2/1 -> Memory1/1, Gain6/1, Integrator2/1
  Divide2/1 -> Add14/2
  Add12/1 -> Product1/2
  Add13/1 -> Gain8/1
  Integrator3/1 -> Add15/1, Gain9/1
  Gain8/1 -> Add8/3
  Constant5/1 -> Mod1/2
  Constant6/1 -> Add10/2
  Gain6/1 -> Goto2/1
  Integrator2/1 -> Mod1/1  "wt"
  Sin1/1 -> Product1/1
  wN1/1 -> Add13/1, Add15/2
  Uabc/1 -> [Uabc]
  Iabc/1 -> [Iabc]
  P/1 -> Subsystem/2(P)
  Pref/1 -> Subsystem/1(Pref)
  Qref/1 -> Subsystem/3(Qref)
  Q/1 -> Subsystem/4(Q)
  From13/1 -> Subsystem1/4(Q)
  From10/1 -> Subsystem1/1(Pref)
  Subsystem1/1(wt) -> Goto11/1
  From11/1 -> Subsystem1/2(P)
  Subsystem1/3(Eabc) -> Goto12/1
  From12/1 -> Subsystem1/3(Qref)
  Subsystem1/2(f) -> Goto10/1
  Subsystem/3(Eabc) -> Eabc/1
  Subsystem/1(wt) -> wt/1
  Subsystem/2(f) -> Scope/1, f/1

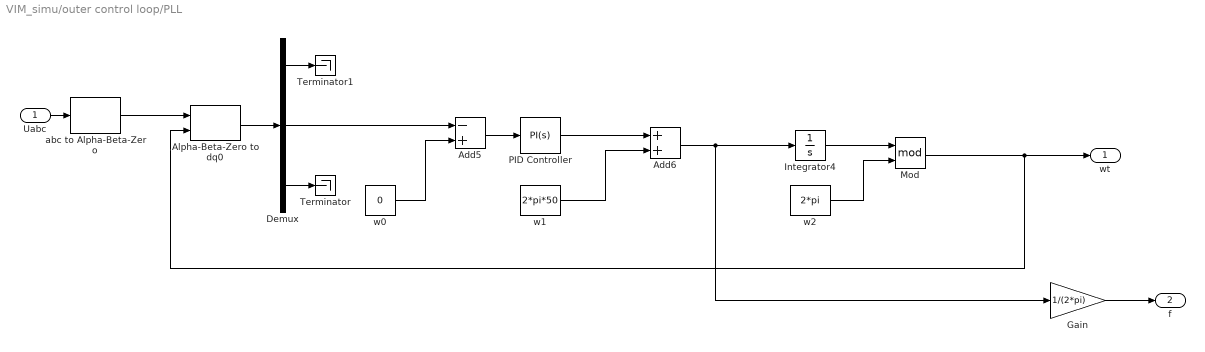
== system VIM_simu/outer control loop/PLL ==
  Uabc : Inport
  Add5 : Sum  Inputs=-+
  Add6 : Sum
  Alpha-Beta-Zero to dq0 : spsAlphaBetaZerotodq0Lib/Alpha-Beta-Zero to dq0  Alignment=90 degrees behind phase A axis
  Demux : Demux  Outputs=3
  Gain : Gain  Gain=1/(2*pi)
  Integrator4 : Integrator
  Mod : Math  Operator=mod
  PID Controller : slpidlib/PID Controller  Controller=PI  Form=Parallel  TimeDomain=Continuous-time  UseExternalTs=off  SampleTime=-1  IntegratorMethod=Forward Euler  FilterMethod=Forward Euler  ControllerParametersSource=internal  P=10  I=50000  UseKiTs=off  D=0  N=100  UseFilter=on  TunerSelectOption=Transfer Function Based (PID Tuner App)  InitialConditionSource=internal  InitialConditionForIntegrator=0  InitialConditionForFilter=0  DifferentiatorICPrevScaledInput=0  ExternalReset=none  TrackingMode=off  Kt=1  LimitOutput=off  SatLimitsSource=internal  UpperSaturationLimit=inf  LowerSaturationLimit=-inf  LinearizeAsGain=on  AntiWindupMode=none  Kb=1  LimitIntegrator=off  UpperIntegratorSaturationLimit=inf  LowerIntegratorSaturationLimit=-inf  POutMin=[]  POutMax=[]  IOutMin=[]  IOutMax=[]  DOutMin=[]  DOutMax=[]  NOutMin=[]  NOutMax=[]  SumOutMin=[]  SumOutMax=[]  SaturationOutMin=[]  SaturationOutMax=[]  PParamMin=[]  PParamMax=[]  IParamMin=[]  IParamMax=[]  DParamMin=[]  DParamMax=[]  NParamMin=[]  NParamMax=[]  KbParamMin=[]  KbParamMax=[]  KtParamMin=[]  KtParamMax=[]  KbOutMin=[]  KbOutMax=[]  KtOutMin=[]  KtOutMax=[]  IntegratorOutMin=[]  IntegratorOutMax=[]  FilterOutMin=[]  FilterOutMax=[]  SumI1OutMin=[]  SumI1OutMax=[]  SumI2OutMin=[]  SumI2OutMax=[]  SumI3OutMin=[]  SumI3OutMax=[]  SumI4OutMin=[]  SumI4OutMax=[]  SumDOutMin=[]  SumDOutMax=[]  DifferentiatorOutMin=[]  DifferentiatorOutMax=[]  FilterDiffOutCoefMin=[]  FilterDiffOutCoefMax=[]  ReciprocalOutMin=[]  ReciprocalOutMax=[]  SumDenOutMin=[]  SumDenOutMax=[]  SumNumOutMin=[]  SumNumOutMax=[]  DivideOutMin=[]  DivideOutMax=[]  UdiffTsProdOutMin=[]  UdiffTsProdOutMax=[]  NTsProdOutMin=[]  NTsProdOutMax=[]  UintegralTsProdOutMin=[]  UintegralTsProdOutMax=[]  UngainTsProdOutMin=[]  UngainTsProdOutMax=[]  ClampingZeroOutDataTypeStr=Inherit: Inherit via back propagation  ClampingZeroOutMin=[]  ClampingZeroOutMax=[]  FilterDenConstantOutDataTypeStr=Inherit: Inherit via back propagation  FilterDenConstantOutMin=[]  FilterDenConstantOutMax=[]  PCopyOutDataTypeStr=Inherit: Inherit via back propagation  PCopyOutMin=[]  PCopyOutMax=[]  NCopyOutDataTypeStr=Inherit: Inherit via back propagation  NCopyOutMin=[]  NCopyOutMax=[]  IntegratorContinuousStateAttributes=''  IntegratorStateMustResolveToSignalObject=off  IntegratorRTWStateStorageClass=Auto  FilterContinuousStateAttributes=''  FilterStateMustResolveToSignalObject=off  FilterRTWStateStorageClass=Auto  ParallelPVariant=InternalParameters  IdealPVariant=Disabled  IVariant=InternalParameters  DVariant=Disabled  IntegratorVariant=Continuous  SatVariant=Disabled  AWVariant=Passthrough  PCopyVariant=Disabled  TRVariant=Disabled  FdbkBlocksVariant=Forward  IdealPFdbkVariant=Disabled  SatFdbkVariant=Disabled  DerivativeFilterVariant=Disabled  NVariant=Disabled  NCopyVariant=Disabled_SignalSpec  FilterICVariant=Disabled  IntegratorICVariant=InternalICs  ExternalResetVariant=Disabled  TRSumVariant=Passthrough  SumFdbkVariant=Disabled  SumVariant=Sum_PI  TsampFilterVariant=InternalTs  TsampNgainVariant=Passthrough  TsampIntegralVariant=Passthrough  ExternalSaturationOutDataTypeStr=Inherit: Same as second input
  Terminator : Terminator
  Terminator1 : Terminator
  abc to Alpha-Beta-Zero : spsabctoAlphaBetaZeroLib/abc to Alpha-Beta-Zero
  w0 : Constant  Value=0
  w1 : Constant  Value=2*pi*50
  w2 : Constant  Value=2*pi
  wt : Outport
  f : Outport  Port=2
  wires:
  Demux/1 -> Terminator1/1
  Demux/2 -> Add5/1
  abc to Alpha-Beta-Zero/1 -> Alpha-Beta-Zero to dq0/1
  Uabc/1 -> abc to Alpha-Beta-Zero/1
  w0/1 -> Add5/2
  Demux/3 -> Terminator/1
  Integrator4/1 -> Mod/1
  Alpha-Beta-Zero to dq0/1 -> Demux/1
  Add5/1 -> PID Controller/1
  w1/1 -> Add6/2
  PID Controller/1 -> Add6/1
  Mod/1 -> wt/1, Alpha-Beta-Zero to dq0/2
  w2/1 -> Mod/2
  Add6/1 -> Gain/1, Integrator4/1
  Gain/1 -> f/1

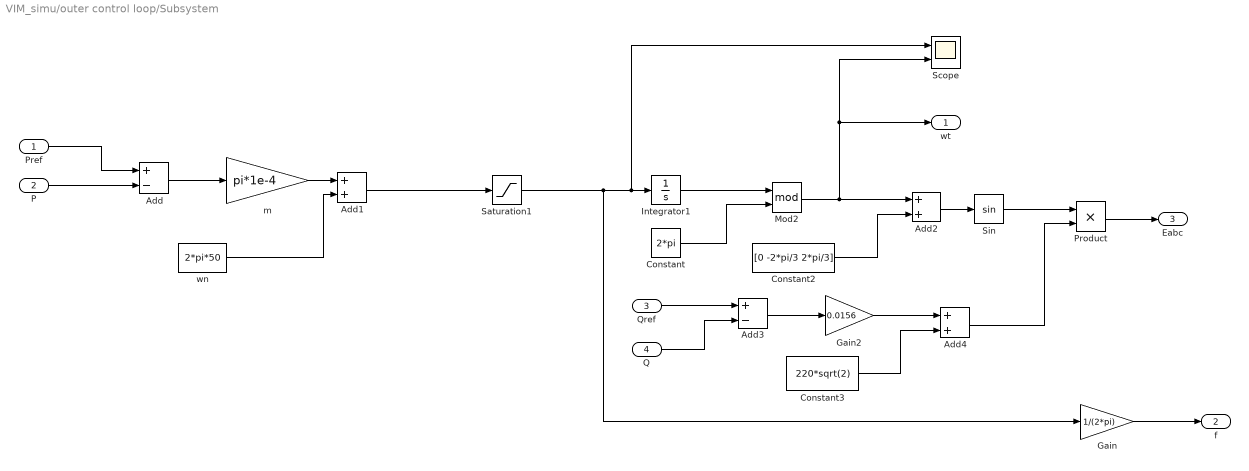
== system VIM_simu/outer control loop/Subsystem ==
  Pref : Inport
  P : Inport  Port=2
  Qref : Inport  Port=3
  Q : Inport  Port=4
  Add : Sum  Inputs=+-
  Add1 : Sum
  Add2 : Sum
  Add3 : Sum  Inputs=+-
  Add4 : Sum
  Constant : Constant  Value=2*pi
  Constant2 : Constant  Value=[0 -2*pi/3 2*pi/3]
  Constant3 : Constant  Value=220*sqrt(2)
  Gain : Gain  Gain=1/(2*pi)
  Gain2 : Gain  Gain=0.0156
  Integrator1 : Integrator
  Mod2 : Math  Operator=mod
  Product : Product
  Saturation1 : Saturate  UpperLimit=2*pi*51  LowerLimit=2*pi*49
  Scope : Scope  NumInputPorts=2
  Sin : Trigonometry
  m : Gain  Gain=pi*1e-4
  wn : Constant  Value=2*pi*50
  wt : Outport
  f : Outport  Port=2
  Eabc : Outport  Port=3
  wires:
  Qref/1 -> Add3/1
  Q/1 -> Add3/2
  Constant2/1 -> Add2/2
  Add2/1 -> Sin/1
  m/1 -> Add1/1
  Add4/1 -> Product/2
  Gain2/1 -> Add4/1
  Integrator1/1 -> Mod2/1
  Sin/1 -> Product/1
  Add/1 -> m/1
  P/1 -> Add/2
  wn/1 -> Add1/2
  Constant3/1 -> Add4/2
  Constant/1 -> Mod2/2
  Mod2/1 -> Add2/1, Scope/2, wt/1
  Add3/1 -> Gain2/1
  Pref/1 -> Add/1
  Gain/1 -> f/1
  Product/1 -> Eabc/1
  Add1/1 -> Saturation1/1
  Saturation1/1 -> Gain/1, Scope/1, Integrator1/1

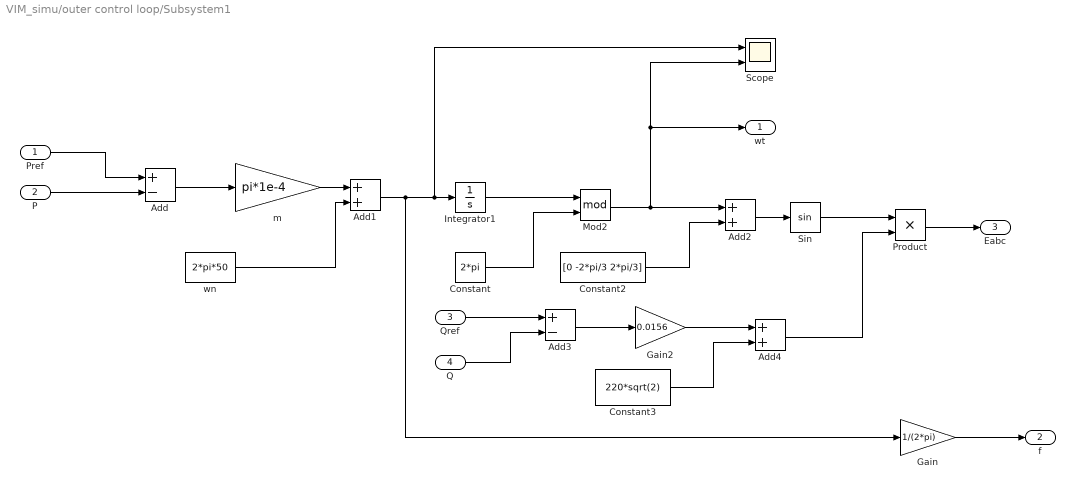
== system VIM_simu/outer control loop/Subsystem1 ==
  Pref : Inport
  P : Inport  Port=2
  Qref : Inport  Port=3
  Q : Inport  Port=4
  Add : Sum  Inputs=+-
  Add1 : Sum
  Add2 : Sum
  Add3 : Sum  Inputs=+-
  Add4 : Sum
  Constant : Constant  Value=2*pi
  Constant2 : Constant  Value=[0 -2*pi/3 2*pi/3]
  Constant3 : Constant  Value=220*sqrt(2)
  Gain : Gain  Gain=1/(2*pi)
  Gain2 : Gain  Gain=0.0156
  Integrator1 : Integrator
  Mod2 : Math  Operator=mod
  Product : Product
  Scope : Scope  NumInputPorts=2
  Sin : Trigonometry
  m : Gain  Gain=pi*1e-4
  wn : Constant  Value=2*pi*50
  wt : Outport
  f : Outport  Port=2
  Eabc : Outport  Port=3
  wires:
  Qref/1 -> Add3/1
  Q/1 -> Add3/2
  Constant2/1 -> Add2/2
  Add2/1 -> Sin/1
  Add1/1 -> Gain/1, Scope/1, Integrator1/1
  m/1 -> Add1/1
  Add4/1 -> Product/2
  Gain2/1 -> Add4/1
  Integrator1/1 -> Mod2/1
  Sin/1 -> Product/1
  Add/1 -> m/1
  P/1 -> Add/2
  wn/1 -> Add1/2
  Constant3/1 -> Add4/2
  Constant/1 -> Mod2/2
  Mod2/1 -> Add2/1, Scope/2, wt/1
  Add3/1 -> Gain2/1
  Pref/1 -> Add/1
  Gain/1 -> f/1
  Product/1 -> Eabc/1

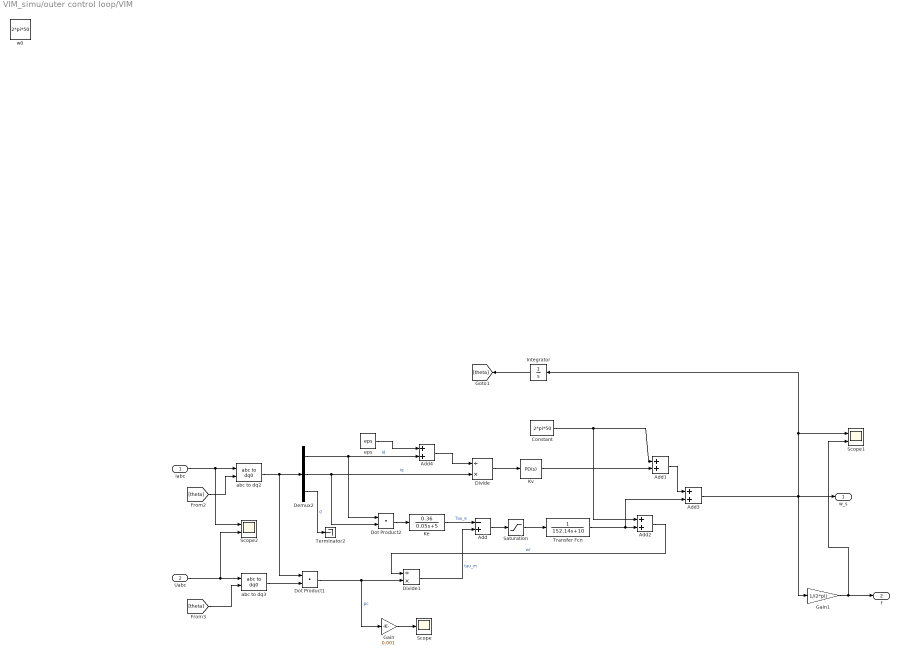
== system VIM_simu/outer control loop/VIM ==
  Iabc : Inport
  Uabc : Inport  Port=2
  Add : Sum  Inputs=-+
  Add{1..4} (4 alike) : Sum
  Constant : Constant  Value=2*pi*50
  Demux2 : Demux  Outputs=3
  Divide : Product  Inputs=/*
  Divide1 : Product  Inputs=/*
  Dot Product1 : DotProduct  OutDataTypeStr=Inherit: Inherit via internal rule
  Dot Product2 : DotProduct  OutDataTypeStr=Inherit: Inherit via internal rule
  Gain : Gain  Gain=0.001
  Gain1 : Gain  Gain=1/(2*pi)
  Integrator : Integrator
  Ke : TransferFcn  Numerator=[0.36]  Denominator=[0.05 5]  ParameterTunability=Optimized
  Kv : slpidlib/PID Controller  Controller=PD  Form=Parallel  TimeDomain=Continuous-time  UseExternalTs=off  SampleTime=-1  IntegratorMethod=Forward Euler  FilterMethod=Forward Euler  ControllerParametersSource=internal  P=0.01  I=1  UseKiTs=off  D=1  N=100  UseFilter=on  TunerSelectOption=Transfer Function Based (PID Tuner App)  InitialConditionSource=internal  InitialConditionForIntegrator=0  InitialConditionForFilter=0  DifferentiatorICPrevScaledInput=0  ExternalReset=none  TrackingMode=off  Kt=1  LimitOutput=off  SatLimitsSource=internal  UpperSaturationLimit=inf  LowerSaturationLimit=-inf  LinearizeAsGain=on  AntiWindupMode=none  Kb=1  LimitIntegrator=off  UpperIntegratorSaturationLimit=inf  LowerIntegratorSaturationLimit=-inf  POutMin=[]  POutMax=[]  IOutMin=[]  IOutMax=[]  DOutMin=[]  DOutMax=[]  NOutMin=[]  NOutMax=[]  SumOutMin=[]  SumOutMax=[]  SaturationOutMin=[]  SaturationOutMax=[]  PParamMin=[]  PParamMax=[]  IParamMin=[]  IParamMax=[]  DParamMin=[]  DParamMax=[]  NParamMin=[]  NParamMax=[]  KbParamMin=[]  KbParamMax=[]  KtParamMin=[]  KtParamMax=[]  KbOutMin=[]  KbOutMax=[]  KtOutMin=[]  KtOutMax=[]  IntegratorOutMin=[]  IntegratorOutMax=[]  FilterOutMin=[]  FilterOutMax=[]  SumI1OutMin=[]  SumI1OutMax=[]  SumI2OutMin=[]  SumI2OutMax=[]  SumI3OutMin=[]  SumI3OutMax=[]  SumI4OutMin=[]  SumI4OutMax=[]  SumDOutMin=[]  SumDOutMax=[]  DifferentiatorOutMin=[]  DifferentiatorOutMax=[]  FilterDiffOutCoefMin=[]  FilterDiffOutCoefMax=[]  ReciprocalOutMin=[]  ReciprocalOutMax=[]  SumDenOutMin=[]  SumDenOutMax=[]  SumNumOutMin=[]  SumNumOutMax=[]  DivideOutMin=[]  DivideOutMax=[]  UdiffTsProdOutMin=[]  UdiffTsProdOutMax=[]  NTsProdOutMin=[]  NTsProdOutMax=[]  UintegralTsProdOutMin=[]  UintegralTsProdOutMax=[]  UngainTsProdOutMin=[]  UngainTsProdOutMax=[]  ClampingZeroOutDataTypeStr=Inherit: Inherit via back propagation  ClampingZeroOutMin=[]  ClampingZeroOutMax=[]  FilterDenConstantOutDataTypeStr=Inherit: Inherit via back propagation  FilterDenConstantOutMin=[]  FilterDenConstantOutMax=[]  PCopyOutDataTypeStr=Inherit: Inherit via back propagation  PCopyOutMin=[]  PCopyOutMax=[]  NCopyOutDataTypeStr=Inherit: Inherit via back propagation  NCopyOutMin=[]  NCopyOutMax=[]  IntegratorContinuousStateAttributes=''  IntegratorStateMustResolveToSignalObject=off  IntegratorRTWStateStorageClass=Auto  FilterContinuousStateAttributes=''  FilterStateMustResolveToSignalObject=off  FilterRTWStateStorageClass=Auto  ParallelPVariant=InternalParameters  IdealPVariant=Disabled  IVariant=Disabled  DVariant=InternalParameters  IntegratorVariant=Disabled  SatVariant=Disabled  AWVariant=Disabled  PCopyVariant=Disabled  TRVariant=Disabled  FdbkBlocksVariant=Forward  IdealPFdbkVariant=Disabled  SatFdbkVariant=Disabled  DerivativeFilterVariant=ContFilter  NVariant=InternalParameters  NCopyVariant=Disabled  FilterICVariant=InternalICsFilter  IntegratorICVariant=Disabled  ExternalResetVariant=Disabled  TRSumVariant=Passthrough  SumFdbkVariant=Disabled  SumVariant=Sum_PD  TsampFilterVariant=InternalTs  TsampNgainVariant=Passthrough  TsampIntegralVariant=Disabled_SignalSpec  ExternalSaturationOutDataTypeStr=Inherit: Same as second input
  Saturation : Saturate  UpperLimit=1  LowerLimit=-1
  Scope : Scope
  Scope1 : Scope  NumInputPorts=2
  Scope2 : Scope  NumInputPorts=2
  Terminator2 : Terminator
  Transfer Fcn : TransferFcn  Denominator=[152.14 10]  ParameterTunability=Optimized
  abc to dq2 : spsabctodq0Lib/abc to dq0  Alignment=90 degrees behind phase A axis
  abc to dq3 : spsabctodq0Lib/abc to dq0  Alignment=90 degrees behind phase A axis
  eps : Constant  Value=eps
  w0 : Constant  Value=2*pi*50
  w_s : Outport
  f : Outport  Port=2
  wires:
  Add2/1 -> Divide1/1  "wr"
  Gain/1 -> Scope/1
  Add4/1 -> Divide/1
  eps/1 -> Add4/1
  Saturation/1 -> Transfer Fcn/1
  Ke/1 -> Add/1  "Tau_e"
  Dot Product1/1 -> Gain/1, Divide1/2  "pc"
  Demux2/3 -> Terminator2/1  "0"
  [theta] -> abc to dq2/2
  [theta] -> abc to dq3/2
  Integrator/1 -> [theta]
  Add1/1 -> Add3/1
  Transfer Fcn/1 -> Add2/2, Add3/2
  Add/1 -> Saturation/1
  Divide1/1 -> Add/2  "tau_m"
  Dot Product2/1 -> Ke/1
  Constant/1 -> Add1/1, Add2/1
  Kv/1 -> Add1/2
  Divide/1 -> Kv/1
  Demux2/2 -> Divide/2, Dot Product2/2  "iq"
  Demux2/1 -> Add4/2, Dot Product2/1  "id"
  abc to dq2/1 -> Demux2/1, Dot Product1/1
  abc to dq3/1 -> Dot Product1/2
  Uabc/1 -> Scope2/2, abc to dq3/1
  Iabc/1 -> Scope2/1, abc to dq2/1
  Gain1/1 -> Scope1/2, f/1
  Add3/1 -> Gain1/1, Integrator/1, Scope1/1, w_s/1

== matlab function VIM_simu/Torque2 ==
  settings: updateMethod=DISCRETE
  data: Ids input double size=[1 1]; Iqs input double size=[1 1]; Vds input double size=[1 1]; Vqs input double size=[1 1]; tau_e output double size=[1 1]; params input Bus: paramsBusTorque; tau_m output double size=[1 1]; delta_omega_r output double size=[1 1]
function [tau_e, tau_m, delta_omega_r] = calculate_virtual_torque(Ids, Iqs, Vds, Vqs, params)
%#codegen
% Inputs:
% Vds - d-axis stator voltage
% Vqs - q-axis stator voltage
% Ids - d-axis stator current
% Iqs - q-axis stator current
% params - structure containing motor parameters
% Outputs:
% tau_e - electromagnetic torque
% tau_m - mechanical torque
% delta_omega_r - change in rotor angular speed

% Extract parameters from the input structure
%Rs = params.Rs;
Rr = params.Rr;
Ls = params.Ls;
Lr = params.Lr;
Lm = params.Lm;
psi_dr = params.psi_dr;
omega0 = params.omega0;
D = params.D;
J = params.J;
delta_omega_r = params.delta_omega_r;

% Calculate stator flux linkages
psi_ds = (Ls - (Lm^2 / Lr)) * Ids + (Lm / Lr) * psi_dr;
psi_qs = (Ls - (Lm^2 / Lr)) * Iqs;

% Calculate electromagnetic torque
tau_e = (3/2) * (Lm / Lr) * psi_dr * Iqs;

% Calculate mechanical torque
Pc = Vds * Ids + Vqs * Iqs; % Output active power
tau_m = Pc / (omega0 + delta_omega_r);

% Calculate change in rotor angular speed
% Use a first-order system to approximate the dynamics
tau_e_freq = (3/2) * (Rr * Lm^2) / (Rr * Lr) * Ids * Iqs; % Simplified frequency domain torque
delta_omega_r = (1 / (J + D)) * (tau_m - tau_e_freq);

% No need to use impulse or tf functions
end

== matlab function VIM_simu/Current2 ==
  settings: updateMethod=DISCRETE
  data: params input Bus: motorParamsBus; Vds input double size=[1 1]; Vqs input double size=[1 1]; idr output double size=[1 1]; iqr output; ids output double size=[1 1]; iqs output double size=[1 1]
function [idr, iqr, ids, iqs] = motorCurrents(params, Vds, Vqs)
% Inputs:
% Vqs - q-axis stator voltage
% Vds - d-axis stator voltage
% params - structure containing motor parameters
% Outputs:
% ids - d-axis stator current
% iqs - q-axis stator current
% idr - d-axis rotor current
% iqr - q-axis rotor current

% Motor parameters
Rs = params.Rs; % Stator resistance
Rr = params.Rr; % Rotor resistance
Ls = params.Ls; % Stator inductance
Lr = params.Lr; % Rotor inductance
Lm = params.Lm; % Mutual inductance
omega_r = params.omega_r; % Rotor angular velocity
omega_s = params.omega_s; % Synchronous angular velocity

% Initialize state variables
persistent lambda_ds lambda_qs lambda_dr lambda_qr;
if isempty(lambda_ds)
    lambda_ds = 0;
    lambda_qs = 0;
    lambda_dr = 0;
    lambda_qr = 0;
end

% Time step (assumed constant for simplicity)
dt = params.dt;


% Calculate stator and rotor currents
ids = (lambda_ds - Lm * lambda_dr) / Ls;
iqs = (lambda_qs - Lm * lambda_qr) / Ls;
idr = (lambda_dr - Lm * ids) / Lr;
iqr = (lambda_qr - Lm * iqs) / Lr;


% Stator flux linkages
lambda_ds = lambda_ds + (Vds - Rs * ids + omega_r * lambda_qs) * dt;
lambda_qs = lambda_qs + (Vqs - Rs * iqs - omega_r * lambda_ds) * dt;

% Rotor flux linkages
lambda_dr = lambda_dr + (-Rr * idr + (omega_s - omega_r) * lambda_qr) * dt;
lambda_qr = lambda_qr + (-Rr * iqr - (omega_s - omega_r) * lambda_dr) * dt;
